simulink model "kalman_try_1"  (R2020a)
settings: Solver=VariableStepAuto  StartTime=0.0  StopTime=10.0  RelTol=1e-3
libraries: audiosources x1, dsparch4 x1, dspadpt3 x1
settings Model: Creator=Karan  LastModifiedBy=Karan

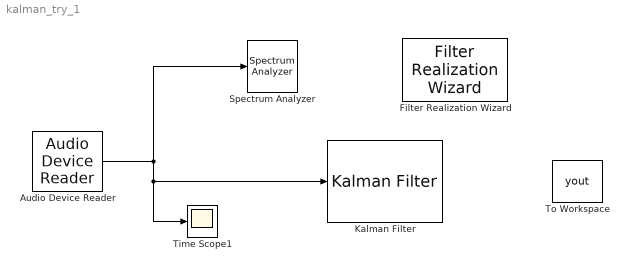
== system kalman_try_1 ==
  Audio Device Reader : audiosources/Audio Device Reader  Driver=DirectSound  Device=Default  SampleRate=44100  NumChannels=1  SamplesPerFrame=1024  BitDepth=16-bit integer  NumBuffers=10  DefaultInputChannelMapping=on  InputChannelMapping=1:2  OutputNumOverrunSamples=off  OutputDataType=double  DriverIdx=1  DeviceWarnFlag=''
      settings: SourceProductBaseCode=AU
  Filter Realization Wizard : dsparch4/Filter Realization Wizard
      settings: SourceProductBaseCode=DS
  Kalman Filter : dspadpt3/Kalman Filter  num_targets=7  sourceEnable=Always  isReset=on  X=zeros([6, 1])  P=10*eye(6)  A=[1 0 1 0 0 0;0 1 0 1 0 0; 0 0 1 0 0 0; 0 0 0 1 0 0; 0 0 0 0 1 0; 0 0 0 0 0 1]  sourceMeasure=Specify via Dialog  H=[1 0 0 0 0 0; 0 1 0 0 0 0; 0 0 0 0 1 0; 0 0 0 0 0 1]  Q=0.05*eye(6)  R=eye(4)  isOutputEstMeasure=off  isOutputEstState=off  isOutputEstError=off  isOutputPrdMeasure=on  isOutputPrdState=off  isOutputPrdError=off
      settings: SourceProductBaseCode=DS
  Spectrum Analyzer : SpectrumAnalyzer
  Time Scope1 : Scope
  To Workspace : ToWorkspace  VariableName=yout  SampleTime=-1
      settings: Save2DSignal=2-D array (concatenate along first dimension)
  wires:
  Audio Device Reader/1 -> Kalman Filter/1, Time Scope1/1, Spectrum Analyzer/1
  ? -> To Workspace/1
